simulink model "Inverter_analysis"  (R2024b)
settings: Solver=VariableStepAuto  StartTime=0.0  StopTime=100  FixedStep=1e-4  RelTol=1e-4
undefined symbols (not defined in the file or in its folder): Frequency, Torque
libraries: spsMosfetLib x4, simulink x2, spsTHDLib x2, spsDCVoltageSourceLib x1, dspfdesign x1, spsCurrentMeasurementLib x1, spsVoltageMeasurementLib x1, spsMultimeterLib x1, spsSeriesRLCBranchLib x1, spsSinglePhaseAsynchronousMachineLib x1, sps_lib x1
settings Model: Creator=Raghav  LastModifiedBy=Raghav

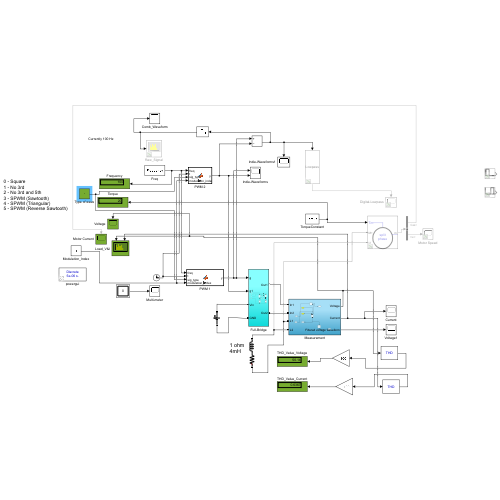
[thumbnail: Simulink's stored preview of the top-level diagram]
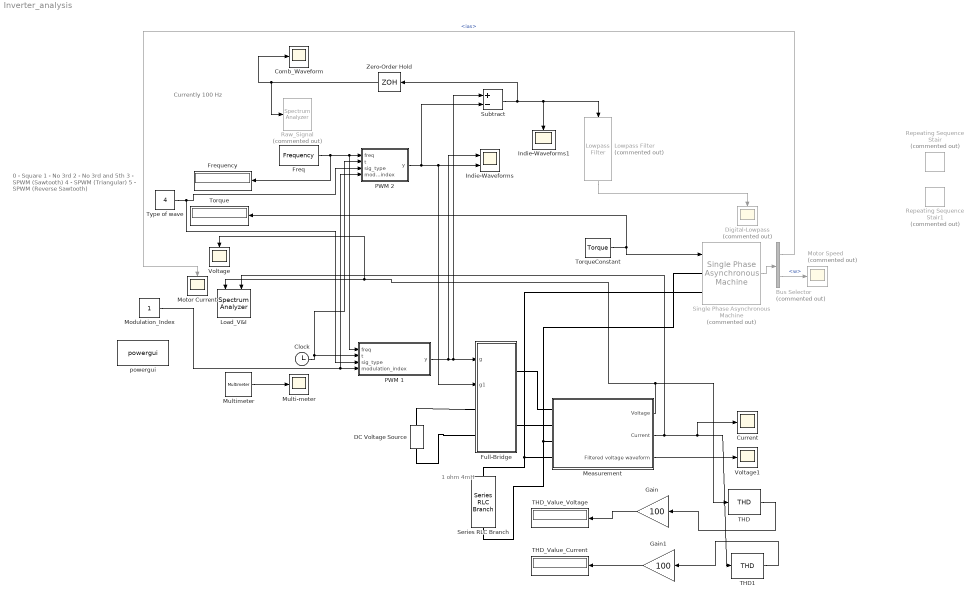
== system Inverter_analysis ==
  note: 1 ohm
      | 4mH
  note: 0 - Square
      | 1 - No 3rd
      | 2 - No 3rd and 5th
      | 3 - SPWM (Sawtooth)
      | 4 - SPWM (Triangular)
      | 5 - SPWM (Reverse Sawtooth)
  note: Currently 100 Hz
  Bus Selector : BusSelector  Commented=on  OutputSignals=ias,w
  Clock : Clock
  Comb_Waveform : Scope
  Current : Scope
  DC Voltage Source : spsDCVoltageSourceLib/DC Voltage Source  Amplitude=100  Measurements=None
  Digital-Lowpass : Scope  Commented=on
  Freq : Constant  Value=Frequency
  Frequency : Display
  Full-Bridge : Subsystem
  Gain : Gain  Gain=100
  Gain1 : Gain  Gain=100
  Indie-Waveforms : Scope  NumInputPorts=2
  Indie-Waveforms1 : Scope
  Load_V&I : SpectrumAnalyzer  NumInputPorts=2  WindowPosition=[0.000000,36.000000,1920.000000,1009.000000,]  Visible=on  ScopeFrameLocation=window  SpectrumType=RMS  PlotAsTwoSidedSpectrum=off  WindowInvariantSamplesPerUpdate=on  NumTapsPerBand=18  FilterSharpness=0.6  StartFrequency=0  StopFrequency=2700  SpectrumUnits=Vrms  FrequencyOffset=[0]  YLimits=[-8.48806383,76.39257444]  ExpandToolstrip=on  SelectedToolstripTab=spectrumAnalyzerToolstrip.channelMeasurementsTab
      settings: OpenAtSimulationStart=off
  Lowpass Filter : dspfdesign/Lowpass Filter  Commented=on  FilterType=FIR  DesignForMinimumOrder=on  FilterOrder=50  PassbandFrequency=100  StopbandFrequency=400  PassbandRipple=0.1  StopbandAttenuation=80  SampleRateMode=Specify on dialog  SampleRate=3000  SimulateUsing=Interpreted execution  roundingMode=Floor  coeffsDataTypeStr=fixdt(1,16)
  Measurement : Subsystem
  Modulation_Index : Constant
  Motor Current : Scope
  Motor Speed : Scope  Commented=on
  Multi-meter : Scope
  Multimeter : spsMultimeterLib/Multimeter  L=1  sel=1  yselected={}  Gain=0  OutputType=Complex  PlotAtSimulationStop=off  PhasorSimulation=off
  PWM 1 : MATLAB Function  TreatAsAtomicUnit=on
  PWM 2 : MATLAB Function  TreatAsAtomicUnit=on
  Raw_Signal : SpectrumAnalyzer  Commented=on  WindowPosition=[0.000000,36.000000,1920.000000,1009.000000,]  ScopeFrameLocation=window  PlotAsTwoSidedSpectrum=off  WindowInvariantSamplesPerUpdate=on  YLimits=[-99.0542746,41.93021131]  ExpandToolstrip=on
      settings: OpenAtSimulationStart=off
  Repeating Sequence Stair : simulink/Sources/Repeating Sequence Stair  Commented=on  OutValues=[0, 1, 1, 1, 1, 0, 0, 0, 0, 0, 0, 0]  tsamp=1/12  OutMin=[]  OutMax=[]  OutDataTypeStr=double  OutputDataTypeScalingMode=double  OutDataType=fixdt(0,8)  ConRadixGroup=Best Precision: Vector-wise  OutScaling=2^-12
  Repeating Sequence Stair1 : simulink/Sources/Repeating Sequence Stair  Commented=on  OutValues=[0, 0, 0, 0, 0, 0, 0, 1, 1, 1, 1, 0]  tsamp=1/12  OutMin=[]  OutMax=[]  OutDataTypeStr=double  OutputDataTypeScalingMode=double  OutDataType=fixdt(0,8)  ConRadixGroup=Best Precision: Vector-wise  OutScaling=2^-12
  Series RLC Branch : spsSeriesRLCBranchLib/Series RLC Branch  LConnTagsString=__new0  RConnTagsString=__new0  BranchType=RL  Resistance=1  Inductance=4e-3  SetiL0=off  InitialCurrent=0  Capacitance=1e-6  Setx0=off  InitialVoltage=0  Measurements=Branch current
  Single Phase Asynchronous Machine : spsSinglePhaseAsynchronousMachineLib/Single Phase Asynchronous Machine  Commented=on  MechanicalLoad=Torque Tm  UNITS=SI  MachineType=Split Phase  MeasurementBus=on  NominalParameters="[ .25*746  110  60]"  MainWindingStator="[2.02  7.4e-3]"  MainWindingRotor="[4.12  5.6e-3]"  MutualInductance=0.1772  AuxiliaryWinding="[7.14  8.5e-3]"  Mechanical="[0.0146  0  2 1.18]"  CapacitorStart="[2  254.7e-6]"  CapacitorRun="[18  21.1e-6]"  DisconnectionSpeed=75  InitialSpeed=0  DataType=SI  TsPowergui=0  TsBlock=-1
      settings: LibrarySourceBlock=|
      | sps_lib/Electrical Machines/Single Phase
      | Asynchronous Machine
  Subtract : Sum  Inputs=+-
  THD : spsTHDLib/THD  Freq=Frequency  Ts=1e-5
  THD1 : spsTHDLib/THD  Freq=Frequency  Ts=1e-5
  THD_Value_Current : Display
  THD_Value_Voltage : Display
  Torque : Display
  TorqueConstant : Constant  Value=Torque
  Type of wave : Constant  Value=4  SampleTime=-1
  Voltage : Scope
  Voltage1 : Scope
  Zero-Order Hold : ZeroOrderHold  SampleTime=1e-5
  powergui : sps_lib/powergui  Priority=1  SimulationMode=Discrete  SampleTime=0.5e-5  frequency=60  Iterations=50  frequencyindice=0  Pbase=100e6  ErrMax=1e-4  UnitsV=kV  UnitsW=MW  buscounter=0  FunctionMessages=off  echomessages=off  EnableUseOfTLC=off  CurrentSourceSwitches=off  DisableSnubberDevices=off  DisableRonSwitches=off  DisableVfSwitches=off  DisplayEquations=off  AutomaticDiscreteSolvers=off  SolverType=Tustin/Backward Euler (TBE)  Interpol=off  ExternalGateDelay=off  methode=off  Ts=100  x0status=blocks  SPID=on  SwTol=0  HookPort=off  NonlinearTolerance=1e-4  nMaxIteration=100  ContinueOnMaxIteration=off  RestoreLinks=warning  ResistiveCurrentMeasurement=off  Frange=[0:2:500]  Ylog=off  Xlog=on  ShowGrid=off  save=off  variable=ZData  structure=0  ZoomFFT=off  StartTime=0.0  cycles=1  DisplayStyle=1  fundamental=60  FreqAxis=off  MaxFrequency=1000  frequencyindicesteady=1  RmsSteady=1  display=off
  wires:
  Bus Selector/1 -> Motor Current/1  "<ias>"
  Multimeter/1 -> Multi-meter/1
  PWM 1/1(y) -> Subtract/1, Full-Bridge/1(g), Indie-Waveforms/1
  Type of wave/1 -> PWM 1/3(sig_type), PWM 2/3(sig_type)
  Clock/1 -> PWM 2/2(t), PWM 1/2(t)
  Freq/1 -> PWM 1/1(freq), PWM 2/1(freq), Frequency/1
  Zero-Order Hold/1 -> Comb_Waveform/1, Raw_Signal/1
  PWM 2/1(y) -> Indie-Waveforms/2, Full-Bridge/2(g1), Subtract/2
  Subtract/1 -> Zero-Order Hold/1, Indie-Waveforms1/1, Lowpass Filter/1
  Lowpass Filter/1 -> Digital-Lowpass/1
  Measurement/3(Filtered voltage waveform) -> Voltage1/1
  Measurement/2(Current) -> THD1/1, Current/1, Load_V&I/2
  TorqueConstant/1 -> Torque/1, Single Phase Asynchronous Machine/1
  Measurement/1(Voltage) -> THD/1, Voltage/1, Load_V&I/1
  Single Phase Asynchronous Machine/1 -> Bus Selector/1
  THD/1 -> Gain/1
  Bus Selector/2 -> Motor Speed/1  "<w>"
  Gain/1 -> THD_Value_Voltage/1
  THD1/1 -> Gain1/1
  Gain1/1 -> THD_Value_Current/1
  Modulation_Index/1 -> PWM 2/4(modulation_index), PWM 1/4(modulation_index)
  connections:
  DC Voltage Source/RConn1 -- Full-Bridge/LConn1
  DC Voltage Source/LConn1 -- Full-Bridge/LConn2
  Full-Bridge/RConn1 -- Measurement/LConn1
  Full-Bridge/RConn2 -- Measurement/LConn2
  Measurement/LConn4 -- Series RLC Branch/RConn1 -- Single Phase Asynchronous Machine/LConn2
  Measurement/LConn3 -- Series RLC Branch/LConn1 -- Single Phase Asynchronous Machine/LConn1

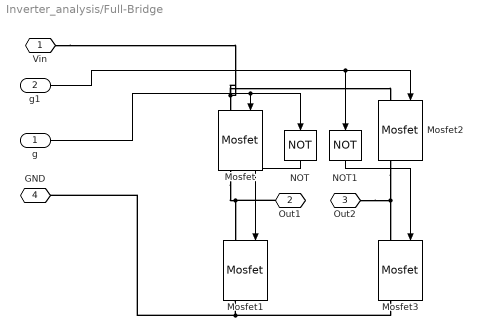
== system Inverter_analysis/Full-Bridge ==
  g : Inport
  g1 : Inport  Port=2
  Mosfet{,1..3} (4 alike) : spsMosfetLib/Mosfet  Ron=0.1  Lon=0  Rd=0.01  Vfd=0  IC=0  Rs=1e5  Cs=inf  Measurements=on
  NOT : Logic  Operator=NOT  IconShape=distinctive  AllPortsSameDT=off  OutDataTypeStr=boolean
  NOT1 : Logic  Operator=NOT  IconShape=distinctive  AllPortsSameDT=off  OutDataTypeStr=boolean
  Vin : PMIOPort  Side=Left
  Out1 : PMIOPort  Port=2  Side=Right
  Out2 : PMIOPort  Port=3  Side=Right
  GND : PMIOPort  Port=4  Side=Left
  wires:
  g/1 -> Mosfet/1, NOT/1
  NOT/1 -> Mosfet1/1
  g1/1 -> Mosfet2/1, NOT1/1
  NOT1/1 -> Mosfet3/1
  connections:
  Mosfet2/RConn1 -- Out2/RConn1 -- Mosfet3/LConn1
  Mosfet/LConn1 -- Vin/RConn1 -- Mosfet2/LConn1
  Mosfet3/RConn1 -- Mosfet1/RConn1 -- GND/RConn1
  Mosfet/RConn1 -- Mosfet1/LConn1 -- Out1/RConn1

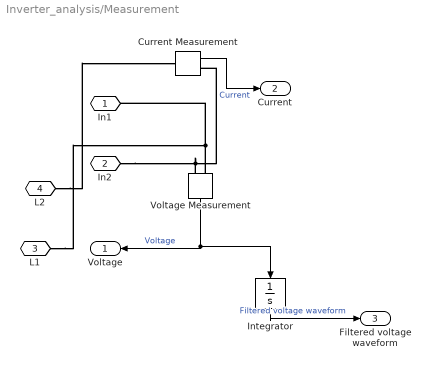
== system Inverter_analysis/Measurement ==
  Current Measurement : spsCurrentMeasurementLib/Current Measurement  PhasorSimulation=off  OutputType=Complex  PSBequivalent=0
  Integrator : Integrator
  Voltage Measurement : spsVoltageMeasurementLib/Voltage Measurement  PhasorSimulation=off  OutputType=Complex  PSBequivalent=0
  In1 : PMIOPort  Side=Left
  In2 : PMIOPort  Port=2  Side=Left
  L1 : PMIOPort  Port=3  Side=Left
  L2 : PMIOPort  Port=4  Side=Left
  Voltage : Outport
  Current : Outport  Port=2
  Filtered voltage waveform : Outport  Port=3
  wires:
  Current Measurement/1 -> Current/1  "Current"
  Voltage Measurement/1 -> Voltage/1, Integrator/1  "Voltage"
  Integrator/1 -> Filtered voltage waveform/1  "Filtered voltage waveform"
  connections:
  In2/RConn1 -- Voltage Measurement/LConn2 -- Current Measurement/RConn1
  Voltage Measurement/LConn1 -- L1/RConn1 -- In1/RConn1
  L2/RConn1 -- Current Measurement/LConn1

== matlab function Inverter_analysis/PWM 2 ==
  data: freq input; y output; t input; sig_type input; modulation_index input
function y = fcn(freq,t, sig_type, modulation_index)
w = 2*pi*freq;
wt = mod(w*t,2*pi);
 %120 mode of conduction
%y = double((wt>=pi)&(wt<=2*pi)); %180 mode of conduction
switch sig_type
    case 1
        y = double((wt>=7*pi/6)&(wt<=11*pi/6)); %120 mode of conduction
    case 2
        y = double((wt>=35*pi/30)&(wt<=39*pi/30)|((wt>=41*pi/30)&(wt<=49*pi/30))|((wt>=51*pi/30)&(wt<=55*pi/30)));
    case 0
        y = double((wt>=pi)&(wt<=2*pi)); %180 mode of conduction
    case 3
        y = LTSPICE_data2(freq,t,0, modulation_index);
    case 4
        y = LTSPICE_data2(freq,t,0.5, modulation_index);
    case 5
        y = LTSPICE_data2(freq,t,1, modulation_index);
    otherwise
        y =0;

end

== matlab function Inverter_analysis/PWM 1 ==
  data: freq input; y output; t input; sig_type input; modulation_index input
function y = fcn(freq,t,sig_type, modulation_index)
w = 2*pi*freq;
wt = mod(w*t,2*pi);
switch sig_type
    case 1
        y = double((wt>=pi/6)&(wt<=5*pi/6)); %120 mode of conduction
        % wavetype = "120 MODE";
    case 2
        y = double((wt>=5*pi/30)&(wt<=9*pi/30)|((wt>=11*pi/30)&(wt<=19*pi/30))|((wt>=21*pi/30)&(wt<=25*pi/30)));
        % wavetype = "3-5 MODE";
    case 0
        y = double((wt>=0)&(wt<=pi)); %180 mode of conduction
        % wavetype = "180 MODE";
    case 3
        y = LTSPICE_data1(freq,t,0, modulation_index);
    case 4
        y = LTSPICE_data1(freq,t,0.5, modulation_index);
    case 5
        y = LTSPICE_data1(freq,t,1, modulation_index);
    otherwise
        y = 0;
        % wavetype = "ERROR";
end
%
